simulink model "bandstop"  (R2016a)
settings: Solver=FixedStepDiscrete  SolverMode=SingleTasking  StartTime=0.0  StopTime=inf  RelTol=1e-3
undefined symbols (not defined in the file or in its folder): fdesignblkfcn, gcbh
libraries: dspsrcs4 x3
settings Model: Creator=Yusuf Khan  LastModifiedBy=Yusuf Khan
settings SolverCC: AutoInsertRateTranBlk=on
settings DataIOCC: LimitDataPoints=on  SaveOutput=off  SignalLogging=off  SaveTime=off
settings DebuggingCC: AlgebraicLoopMsg=error  SingleTaskRateTransMsg=error  AllowSymbolicDim=off
settings ConfigComp: CovModelRefEnable=Off  CovSFcnEnable=off

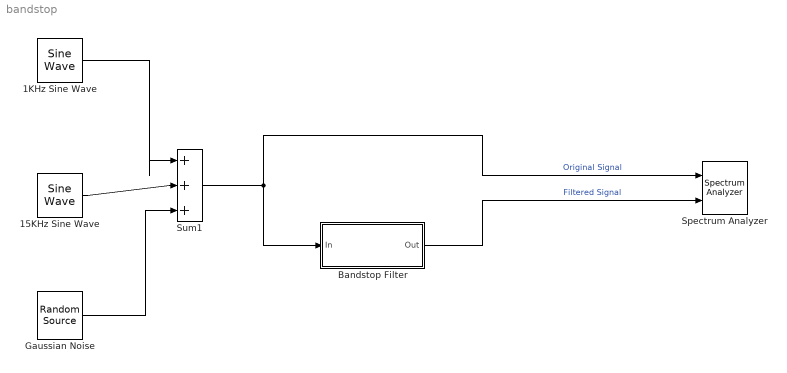
== system bandstop ==
  15KHz Sine Wave : dspsrcs4/Sine Wave  Amplitude=1  Frequency=15000  Phase=0  SampleMode=Discrete  OutComplex=Real  CompMethod=Trigonometric fcn  TableSize=Speed  SampleTime=1/44100  SamplesPerFrame=256  ResetState=Restart at time zero  OutputFrames=off  dataType=double  wordLen=16  udDataType=sfix(16)  fracBitsMode=Best precision  numFracBits=15  OutDataTypeStr=double  LastOutDataTypeStr=double
  1KHz Sine Wave : dspsrcs4/Sine Wave  Amplitude=1  Frequency=1000  Phase=0  SampleMode=Discrete  OutComplex=Real  CompMethod=Trigonometric fcn  TableSize=Speed  SampleTime=1/44100  SamplesPerFrame=256  ResetState=Restart at time zero  OutputFrames=off  dataType=double  wordLen=16  udDataType=sfix(16)  fracBitsMode=Best precision  numFracBits=15  OutDataTypeStr=double  LastOutDataTypeStr=double
  Bandstop Filter : Subsystem  DialogController=fdesignblkfcn  InitFcn=fdesignblkfcn(gcbh, {'InitFcn'});  mask(Bandstop Filter){}
      mask help: Design a bandstop filter
      settings: CopyFcn=fdesignblkfcn(gcbh, {'CopyFcn'});
      mask Help: helpview(mapfilelocation('dsp'), 'dspbandstopfilter');
      mask Display: disp('Bandstop');
  Gaussian Noise : dspsrcs4/Random Source  SrcType=Gaussian  NormMethod=Ziggurat  CltLength=12  MinVal=0  MaxVal=1  MeanVal=0  VarVal=.05  RepMode=Specify seed  rawSeed=1234567  IsInherit=off  SampMode=Discrete  SampTime=1/44100  SampFrame=256  DataType=Double  OutComplex=Real  OutputFrames=off
  Spectrum Analyzer : SpectrumAnalyzer  NumInputPorts=2
  Sum1 : Sum  Inputs=|+++
  wires:
  1KHz Sine Wave/1 -> Sum1/1
  15KHz Sine Wave/1 -> Sum1/2
  Sum1/1 -> Bandstop Filter/1(In), Spectrum Analyzer/1  "Original Signal"
  Bandstop Filter/1(Out) -> Spectrum Analyzer/2  "Filtered Signal"
  Gaussian Noise/1 -> Sum1/3

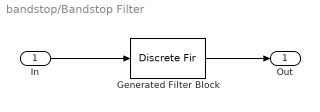
== system bandstop/Bandstop Filter ==
  In : Inport
  Generated Filter Block : DiscreteFir  Tag=BlockMethodSubSystem  Coefficients=[-0.00049984690227429984 9.5100318057543079e-05 -0.018778888889124077 0.00020561736622359334 0.0019605411941897403 0.00023848464356728024 0.011427768692371167 0.00024928020776836409 -0.02634414346835514 0.00022323473160409515 0.033802321854575927 0.00024455404571686537 -0.019823660150559162 0.0002437704533452736 -0.019896328302991071 0.00022786848806519958 0.082714162332195681 0.00025656261277871015 -0.15101859373265938 0.00022072984516976232 0.20526035643478208 0.000247613686607299 0.77489283142488308 0.000247613686607299 0.20526035643478208 0.00022072984516976232 -0.15101859373265938 0.00025656261277871015 0.082714162332195681 0.00022786848806519958 -0.019896328302991071 0.0002437704533452736 -0.019823660150559162 0.00024455404571686537 0.033802321854575927 0.00022323473160409515 -0.02634414346835514 0.00024928020776836409 0.011427768692371167 0.00023848464356728024 0.0019605411941897403 0.00020561736622359334 -0.018778888889124077 9.5100318057543079e-05 -0.00049984690227429984]  InputProcessing=Columns as channels (frame based)
  Out : Outport
  wires:
  Generated Filter Block/1 -> Out/1
  In/1 -> Generated Filter Block/1
